simulink model "Project2eLin"  (R2015b)
settings: Solver=ode5  StartTime=0.0  StopTime=5  FixedStep=0.001  RelTol=1e-3
values from neighbouring files (symbols this model uses):
  c0 = [0;0]    [Project2full.m]
  xss = [x10ss;x20ss]    [Project2full.m]
undefined symbols (not defined in the file or in its folder): A, B, C, D
settings Model: Creator=Dell  LastModifiedBy=Dell
settings DataIOCC: LimitDataPoints=off  TimeSaveName=tout1

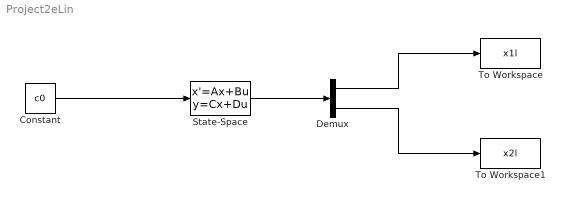
== system Project2eLin ==
  Constant : Constant  Value=c0
  Demux : Demux  Outputs=2
  State-Space : StateSpace  A=A  B=B  C=C  D=D  X0=xss
  To Workspace : ToWorkspace  VariableName=x1l  SampleTime=-1
  To Workspace1 : ToWorkspace  VariableName=x2l  SampleTime=-1
  wires:
  Constant/1 -> State-Space/1
  State-Space/1 -> Demux/1
  Demux/1 -> To Workspace/1
  Demux/2 -> To Workspace1/1
